simulink model "cartpendkalman"  (R2018a)
settings: Solver=VariableStepAuto  StartTime=0.0  StopTime=75  RelTol=1e-3
InitFcn:
  | INITKF
values from neighbouring files (symbols this model uses):
  C = [1 0 0 0]    [INIT.m]    (also in INITKF.m; INITexp.m; INITnonmpc.m)
  K = lqr(A,B,Q,R)    [INIT.m]    (also in INITKF.m; INITexp.m; INITnonmpc.m)
  sysKf = ss(A-Kf*C,[B Kf],eye(4),0*[B Kf])    [INIT.m]    (also in INITKF.m; INITexp.m; INITnonmpc.m)
libraries: dspsrcs4 x3, powerlib_meascontrol x1
settings Model: Creator=Prodigio  LastModifiedBy=Prodigio

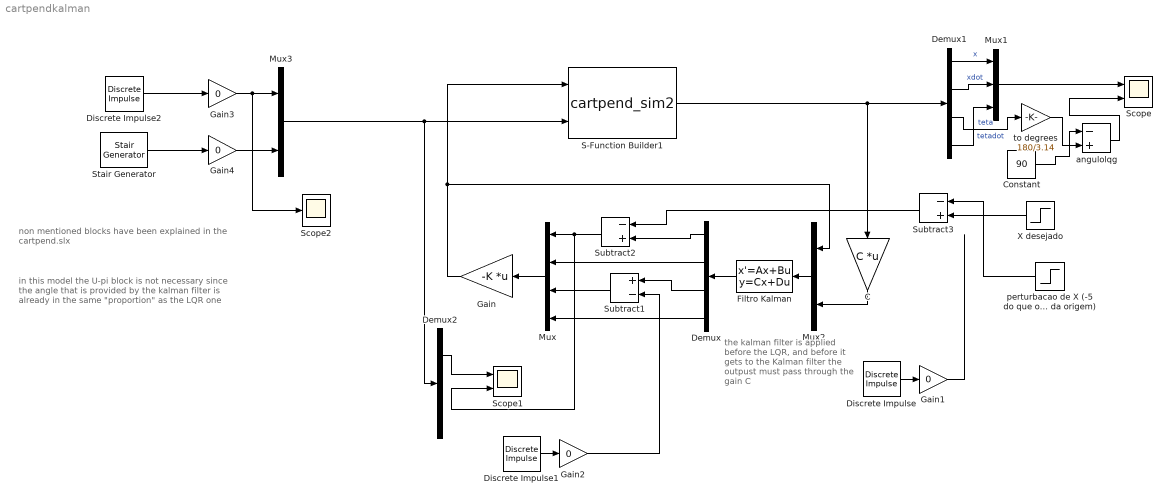
== system cartpendkalman ==
  note: non mentioned blocks have been explained in the cartpend.slx
  note: the kalman filter is applied before the LQR, and before it gets to the Kalman filter the outpust must pass through the gain C
  note: in this model the U-pi block is not necessary since the angle that is provided by the kalman filter is already in the same "proportion" as the LQR one
  C : Gain  Gain=C  Multiplication=Matrix(K*u) (u vector)
  Constant : Constant  Value=90
  Demux : Demux
  Demux1 : Demux
  Demux2 : Demux  Outputs=2
  Discrete Impulse : dspsrcs4/Discrete  Impulse  Delay=10  SampleTime=3  FrameSample=1  OutputFrames=off  dataType=double  isSigned=on  wordLen=16  udDataType=sfix(16)  fracBitsMode=Best precision  numFracBits=15  OutDataTypeStr=double  LastOutDataTypeStr=double
  Discrete Impulse1 : dspsrcs4/Discrete  Impulse  Delay=20  SampleTime=1  FrameSample=1  OutputFrames=off  dataType=double  isSigned=on  wordLen=16  udDataType=sfix(16)  fracBitsMode=Best precision  numFracBits=15  OutDataTypeStr=double  LastOutDataTypeStr=double
  Discrete Impulse2 : dspsrcs4/Discrete  Impulse  Delay=15  SampleTime=3  FrameSample=1  OutputFrames=off  dataType=double  isSigned=on  wordLen=16  udDataType=sfix(16)  fracBitsMode=Best precision  numFracBits=15  OutDataTypeStr=double  LastOutDataTypeStr=double
  Filtro Kalman : StateSpace  A=sysKf.a  B=sysKf.b  C=sysKf.c  D=sysKf.d  InitialCondition=[0 0 0 0]
  Gain : Gain  Gain=-K  Multiplication=Matrix(K*u) (u vector)
  Gain{1..4} (4 alike) : Gain  Gain=0
  Mux : Mux
  Mux1 : Mux  Inputs=3
  Mux2 : Mux  Inputs=2
  Mux3 : Mux  Inputs=2
  S-Function Builder1 : S-Function  InitFcn=try, set_param(gcb,'FunctionName','cartpend_sim2'), end  FunctionName=cartpend_sim2  SFunctionModules=cartpend_sim2_wrapper  SFunctionDeploymentMode=off  EnableBusSupport=off  mask(S-Function Builder){}
      mask help: Simulink:masks:SFunctionBuilder_MD
      mask init:
      | val = [[.9  0.75 0.75 1 1 .9 .9 1]',[1 1 0.75 0.75 .9 .9 1 .9]'];try , sys = get_param(gcb,'SfunBuilderFcnName');if isempty(sys), sys = get_param(gcb,'FunctionName'); end,catch, sys = get_param(gcb,'FunctionName'); end
      settings: CopyFcn=set_param(gcbh,'LinkStatus','none')  PreSaveFcn=try, set_param(gcb,'FunctionName','cartpend_sim2'), end  OpenFcn=sfunctionwizard(gcbh)
      mask Display: plot(val(:,1),val(:,2)),disp(sys), port_label('input',1,'u0'), port_label('input',2,'pert'), port_label('output',1,'y0')
  Scope : Scope  NumInputPorts=2
  Scope1 : Scope  NumInputPorts=2
  Scope2 : Scope
  Stair Generator : powerlib_meascontrol/Pulse & Signal Generators/Stair Generator  t=[15,18, 30,32, 50,52]  e=[-0.4,0, 0.3,0, 0.7,0]  Ts=0
      settings: SourceProductName=Simscape Power Systems
  Subtract1 : Sum  Inputs=+-
  Subtract2 : Sum  Inputs=-+
  Subtract3 : Sum  Inputs=-+
  "X desejado " : Step  Time=15  After=2  SampleTime=0
  angulolqg : Sum  Inputs=-+
  "perturbacao de X (-5 do que onde está, nao da da origem)" : Step  Time=40  After=3  SampleTime=0
  to degrees : Gain  Gain=180/3.14
  wires:
  Gain/1 -> Mux2/1, S-Function Builder1/1
  S-Function Builder1/1 -> Demux1/1, C/1
  Demux1/1 -> Mux1/1  "x"
  Demux1/2 -> Mux1/2  "xdot"
  Demux1/4 -> Mux1/3  "tetadot"
  Demux/2 -> Mux/2
  "X desejado "/1 -> Subtract3/2
  Mux/1 -> Gain/1
  Mux1/1 -> Scope/1
  Demux/3 -> Subtract1/1
  Subtract1/1 -> Mux/3
  Subtract2/1 -> Mux/1, Scope1/2
  Demux/1 -> Subtract2/2
  Subtract3/1 -> Subtract2/1
  Discrete Impulse/1 -> Gain1/1
  Gain2/1 -> Subtract1/2
  Discrete Impulse1/1 -> Gain2/1
  Demux/4 -> Mux/4
  Demux2/1 -> Scope1/1
  Discrete Impulse2/1 -> Gain3/1
  Gain3/1 -> Scope2/1, Mux3/1
  Mux3/1 -> S-Function Builder1/2, Demux2/1
  Stair Generator/1 -> Gain4/1
  Gain4/1 -> Mux3/2
  Demux1/3 -> to degrees/1  "teta"
  to degrees/1 -> angulolqg/2
  angulolqg/1 -> Scope/2
  Constant/1 -> angulolqg/1
  Mux2/1 -> Filtro Kalman/1
  C/1 -> Mux2/2
  Filtro Kalman/1 -> Demux/1
  "perturbacao de X (-5 do que onde está, nao da da origem)"/1 -> Subtract3/1
  Gain1/1 -> ?
  ? -> ?
